simulink library "Bias"  (R2018a)
settings: Solver=VariableStepAuto  StartTime=0.0  StopTime=10.0  RelTol=1e-3
values from neighbouring files (symbols this model uses):
  Ts = 0.01    [Kalman_Filter_Simulink_Example_params.m]
libraries: simulink x3
settings Model: Creator=hussein  LastModifiedBy=hussein

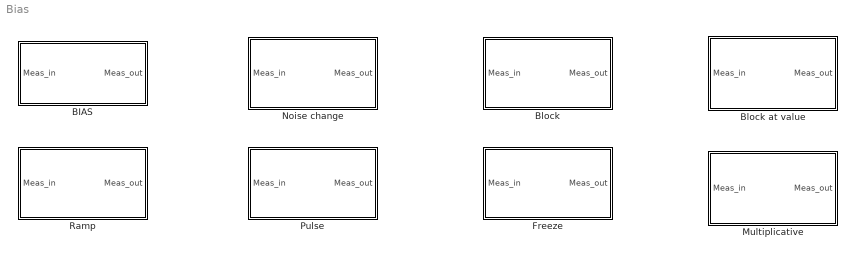
== system Bias ==
  BIAS : Subsystem  mask{Bias=0, Time=0}
      mask prompts: Bias "Bias Value"
      mask init:
      | if(Time<0)
      |     Time=0;
      | end
      mask Help: Bias
      mask Display:
      | disp("Bias");
      | port_label('input',1,'In');
      | port_label('output',1,'Out');
  Block : Subsystem  mask{Noise=0, Time=0}
      mask prompts: Noise "Noise Value"
      mask Display:
      | disp('Block');
      | port_label('input',1,'In');
      | port_label('output',1,'Out');
  Block at value : Subsystem  mask{Value=0, Time=0}
      mask Display:
      | disp('Freeze Value');
      | port_label('input',1,'In');
      | port_label('output',1,'Out');
  Freeze : Subsystem  mask{Time=0}
      mask Display:
      | disp('freeze');
      | port_label('input',1,'In');
      | port_label('output',1,'Out');
  Multiplicative : Subsystem  mask{Gain=0, Time=0}
      mask Display:
      | disp('Mult');
      | port_label('input',1,'In');
      | port_label('output',1,'Out');
  Noise change : Subsystem  mask{Noise_add=0, Time=0}
      mask prompts: Noise_add "Noise Value"
      mask Display:
      | disp('Add Noise');
      | port_label('input',1,'In');
      | port_label('output',1,'Out');
  Pulse : Subsystem  mask{Pulse_value=0.1, Pulse_periode=0, Pulse_width=0, Time=0}
      mask prompts: Pulse_value "Pulse Amp"; Pulse_periode "Periode"; Pulse_width "Pulse width"
      mask init:
      | if(Pulse_value<=0)
      |     Pulse_value=0.1;
      | end
      | if(Pulse_periode<=0)
      |     Pulse_periode=4;
      | end
      | 
      | if(Pulse_width<=0)
      |     Pulse_width=1;
      | end
      mask Display:
      | disp('Pulse');
      | port_label('input',1,'In');
      | port_label('output',1,'Out');
  Ramp : Subsystem  mask{Slope=0, Time=0}
      mask prompts: Slope "Slope Value"
      mask Display:
      | disp('Ramp');
      | port_label('input',1,'In');
      | port_label('output',1,'Out');

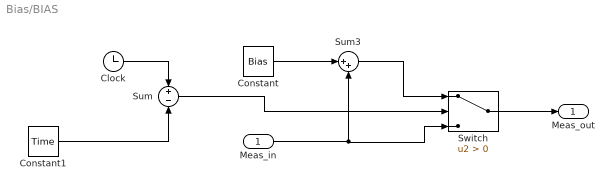
== system Bias/BIAS ==
  "Meas_in " : Inport
  Clock : Clock
  Constant : Constant  Value=Bias
  Constant1 : Constant  Value=Time
  Sum : Sum  Inputs=+-
  Sum3 : Sum  Inputs=|++
  Switch : Switch  Criteria=u2 > Threshold
  Meas_out : Outport
  wires:
  Constant1/1 -> Sum/2
  Sum/1 -> Switch/2
  "Meas_in "/1 -> Sum3/2, Switch/3
  Switch/1 -> Meas_out/1
  Constant/1 -> Sum3/1
  Clock/1 -> Sum/1
  Sum3/1 -> Switch/1

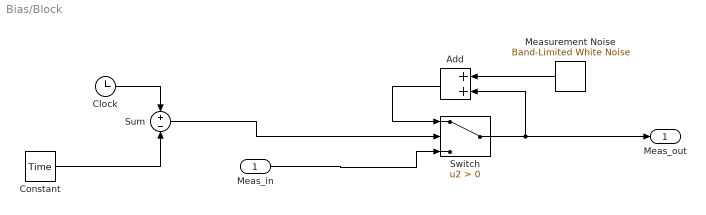
== system Bias/Block ==
  "Meas_in " : Inport
  Add : Sum
  Clock : Clock
  Constant : Constant  Value=Time
  Measurement Noise : simulink/Sources/Band-Limited White Noise  Cov=Noise  Ts=Ts  seed=[12347]
  Sum : Sum  Inputs=+-
  Switch : Switch  Criteria=u2 > Threshold
  Meas_out : Outport
  wires:
  "Meas_in "/1 -> Switch/3
  Constant/1 -> Sum/2
  Switch/1 -> Add/2, Meas_out/1
  Clock/1 -> Sum/1
  Sum/1 -> Switch/2
  Add/1 -> Switch/1
  Measurement Noise/1 -> Add/1

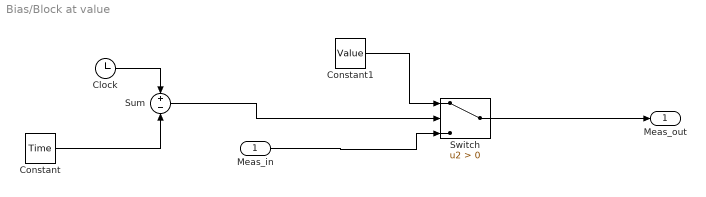
== system Bias/Block at value ==
  "Meas_in " : Inport
  Clock : Clock
  Constant : Constant  Value=Time
  Constant1 : Constant  Value=Value
  Sum : Sum  Inputs=+-
  Switch : Switch  Criteria=u2 > Threshold
  Meas_out : Outport
  wires:
  "Meas_in "/1 -> Switch/3
  Constant/1 -> Sum/2
  Clock/1 -> Sum/1
  Sum/1 -> Switch/2
  Switch/1 -> Meas_out/1
  Constant1/1 -> Switch/1

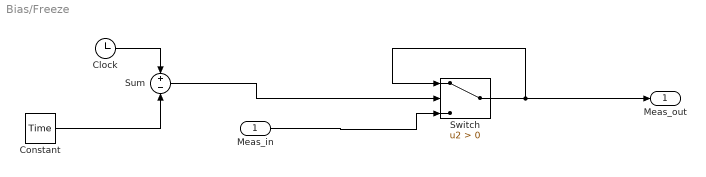
== system Bias/Freeze ==
  "Meas_in " : Inport
  Clock : Clock
  Constant : Constant  Value=Time
  Sum : Sum  Inputs=+-
  Switch : Switch  Criteria=u2 > Threshold
  Meas_out : Outport
  wires:
  Switch/1 -> Switch/1, Meas_out/1
  Sum/1 -> Switch/2
  Clock/1 -> Sum/1
  Constant/1 -> Sum/2
  "Meas_in "/1 -> Switch/3

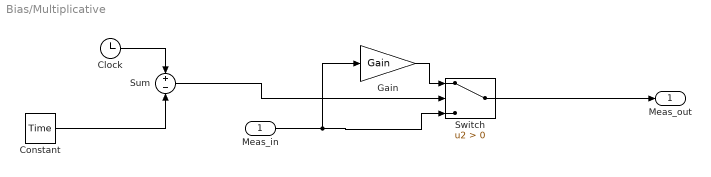
== system Bias/Multiplicative ==
  "Meas_in " : Inport
  Clock : Clock
  Constant : Constant  Value=Time
  Gain : Gain  Gain=Gain
  Sum : Sum  Inputs=+-
  Switch : Switch  Criteria=u2 > Threshold
  Meas_out : Outport
  wires:
  Switch/1 -> Meas_out/1
  Sum/1 -> Switch/2
  Clock/1 -> Sum/1
  Constant/1 -> Sum/2
  "Meas_in "/1 -> Gain/1, Switch/3
  Gain/1 -> Switch/1

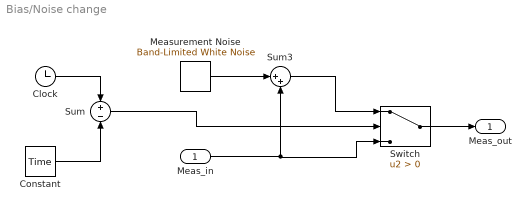
== system Bias/Noise change ==
  "Meas_in " : Inport
  Clock : Clock
  Constant : Constant  Value=Time
  Measurement Noise : simulink/Sources/Band-Limited White Noise  Cov=Noise_add  Ts=Ts  seed=[12347]
  Sum : Sum  Inputs=+-
  Sum3 : Sum  Inputs=|++
  Switch : Switch  Criteria=u2 > Threshold
  Meas_out : Outport
  wires:
  "Meas_in "/1 -> Switch/3, Sum3/2
  Measurement Noise/1 -> Sum3/1
  Sum3/1 -> Switch/1
  Switch/1 -> Meas_out/1
  Clock/1 -> Sum/1
  Sum/1 -> Switch/2
  Constant/1 -> Sum/2

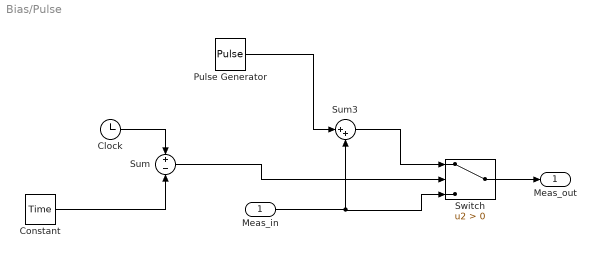
== system Bias/Pulse ==
  "Meas_in " : Inport
  Clock : Clock
  Constant : Constant  Value=Time
  Pulse Generator : DiscretePulseGenerator  Amplitude=Pulse_value  Period=Pulse_periode  PulseWidth=Pulse_width  SampleTime=Ts
  Sum : Sum  Inputs=+-
  Sum3 : Sum  Inputs=|++
  Switch : Switch  Criteria=u2 > Threshold
  Meas_out : Outport
  wires:
  Sum/1 -> Switch/2
  Clock/1 -> Sum/1
  Switch/1 -> Meas_out/1
  Constant/1 -> Sum/2
  Sum3/1 -> Switch/1
  Pulse Generator/1 -> Sum3/1
  "Meas_in "/1 -> Sum3/2, Switch/3

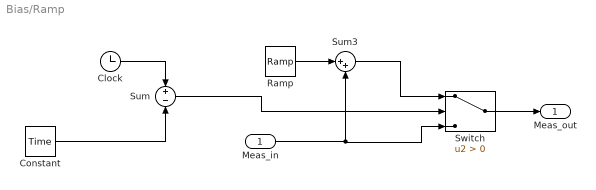
== system Bias/Ramp ==
  "Meas_in " : Inport
  Clock : Clock
  Constant : Constant  Value=Time
  Ramp : simulink/Sources/Ramp  slope=Slope  start=Time  InitialOutput=0
  Sum : Sum  Inputs=+-
  Sum3 : Sum  Inputs=|++
  Switch : Switch  Criteria=u2 > Threshold
  Meas_out : Outport
  wires:
  Sum/1 -> Switch/2
  Clock/1 -> Sum/1
  Switch/1 -> Meas_out/1
  Constant/1 -> Sum/2
  Sum3/1 -> Switch/1
  Ramp/1 -> Sum3/1
  "Meas_in "/1 -> Sum3/2, Switch/3
